simulink model "atmos"  (Simulink 7.5)
settings: Solver=ode45  StartTime=0.0  StopTime=10.0  RelTol=1e-3
settings Model: Creator=knightofaccess  LastModifiedBy=knightofaccess

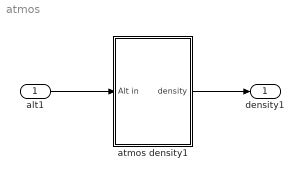
== system atmos ==
  alt1 : Inport  OutDataType=sfix(16)  OutScaling=2^0
  atmos density1 : Subsystem
  density1 : Outport  OutDataType=sfix(16)  OutScaling=2^0
  wires:
  atmos density1/1(density) -> density1/1
  alt1/1 -> atmos density1/1(Alt in)

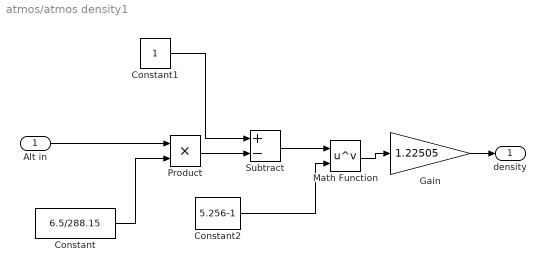
== system atmos/atmos density1 ==
  Alt in : Inport  OutDataType=sfix(16)  OutScaling=2^0
  Constant : Constant  Value=6.5/288.15  OutDataType=sfix(16)  OutScaling=2^0
  Constant1 : Constant  OutDataType=sfix(16)  OutScaling=2^0
  Constant2 : Constant  Value=5.256-1  OutDataType=sfix(16)  OutScaling=2^0
  Gain : Gain  Gain=1.22505  ParameterDataType=sfix(16)  ParameterScaling=2^0  OutDataType=sfix(16)  OutScaling=2^0
  Math Function : Math  Operator=pow  OutDataType=sfix(16)  OutScaling=2^0  SaturateOnIntegerOverflow=on
  Product : Product  OutDataType=sfix(16)  OutScaling=2^0  RndMeth=Zero
  Subtract : Sum  Inputs=+-  OutDataType=sfix(16)  OutScaling=2^-10
  density : Outport  OutDataType=sfix(16)  OutScaling=2^0
  wires:
  Constant/1 -> Product/2
  Product/1 -> Subtract/2
  Constant1/1 -> Subtract/1
  Subtract/1 -> Math Function/1
  Constant2/1 -> Math Function/2
  Math Function/1 -> Gain/1
  Alt in/1 -> Product/1
  Gain/1 -> density/1
